simulink model "notchfilter"  (R2013a)
settings: Solver=ode4  StartTime=0.0  StopTime=1  FixedStep=1e-4  RelTol=1e-3
settings Model: Creator=ugurm  LastModifiedBy=ugurm

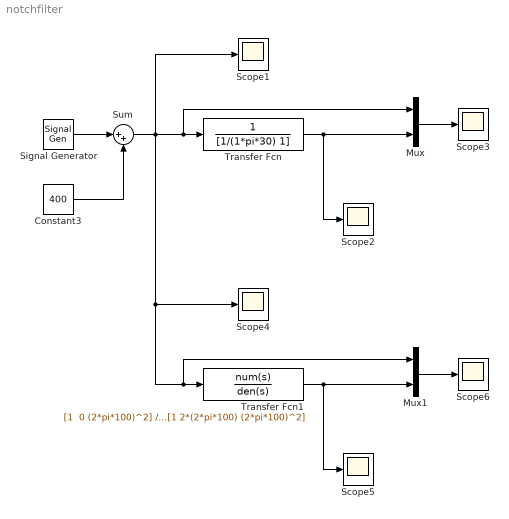
== system notchfilter ==
  Constant3 : Constant  Value=400
  Mux : Mux  Inputs=2
  Mux1 : Mux  Inputs=2
  Scope{1..6} (6 alike) : Scope
      Scope1 settings: YMin=0  YMax=430
      Scope2 settings: YMin=0  YMax=430
      Scope3 settings: YMin=0  YMax=430  SaveName=ScopeData2
      Scope4 settings: YMin=0  YMax=430  SaveName=ScopeData3
      Scope5 settings: YMin=0  YMax=430  SaveName=ScopeData4
      Scope6 settings: YMin=0  YMax=430  SaveName=ScopeData5
  Signal Generator : SignalGenerator  Amplitude=10  Frequency=100
  Sum : Sum  Inputs=|++
  Transfer Fcn : TransferFcn  Denominator=[1/(1*pi*30) 1]
  Transfer Fcn1 : TransferFcn  Numerator="[1  0 (2*pi*100)^2]"  Denominator=[1 2*(2*pi*100) (2*pi*100)^2]
  wires:
  Signal Generator/1 -> Sum/1
  Constant3/1 -> Sum/2
  Transfer Fcn/1 -> Mux/2, Scope2/1
  Mux/1 -> Scope3/1
  Transfer Fcn1/1 -> Mux1/2, Scope5/1
  Mux1/1 -> Scope6/1
  Sum/1 -> Mux1/1, Transfer Fcn1/1, Scope4/1, Mux/1, Transfer Fcn/1, Scope1/1
